simulink model "assembly_a"  (R2021a)
settings: Solver=VariableStepAuto  StartTime=0.0  StopTime=10.0  RelTol=1e-3
values from neighbouring files (symbols this model uses):
  trim_state_lo = [0 0 15000 0 0.0779375118365 0 500 0.0779375118365 0 0 0 0]    [15000_500_lin.mat]    (also in 20000_600_lin.mat = [0 0 20000 0 0.0594178286879 0 600 0.0594178286879 0 0 0 0]; 20000_700_lin.mat = [0 0 20000 0 0.0369748641994 0 700 0.0369748641994 0 0 0 0]; 20000_900_lin.mat = [0 0 20000 0 0.0123475459982 0 900 0.0123475459982 0 0 0 0]; chapter8.mat = [0 0 5000 0 0.182405640343 0 300 0.182405640343 0 0 0 0])
settings Model: Creator=wardb  LastModifiedBy=wardb

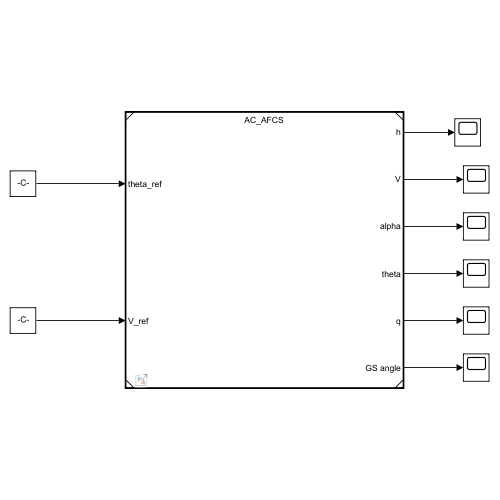
[thumbnail: Simulink's stored preview of the top-level diagram]
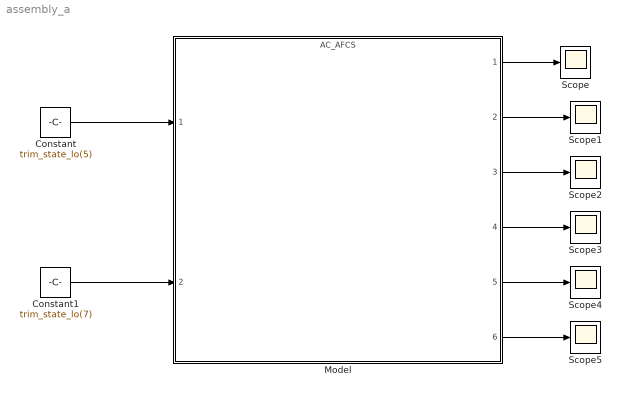
== system assembly_a ==
  Constant : Constant  Value=trim_state_lo(5)
  Constant1 : Constant  Value=trim_state_lo(7)
  Model : ModelReference  ModelNameDialog=AC_AFCS.slx  SimulationMode=Normal  ModelReferenceVersion=4.7
  Scope{,1..5} (6 alike) : Scope
  wires:
  Model/6 -> Scope5/1
  Model/5 -> Scope4/1
  Model/4 -> Scope3/1
  Model/3 -> Scope2/1
  Model/2 -> Scope1/1
  Model/1 -> Scope/1
  Constant/1 -> Model/1
  Constant1/1 -> Model/2
